simulink model "exercises_check"  (R2024a)
settings: Solver=FixedStepAuto  StartTime=0.0  StopTime=100  FixedStep=0.0001  MaxStep=1e-4  RelTol=1e-6
settings Model: Creator=kit  LastModifiedBy=kit

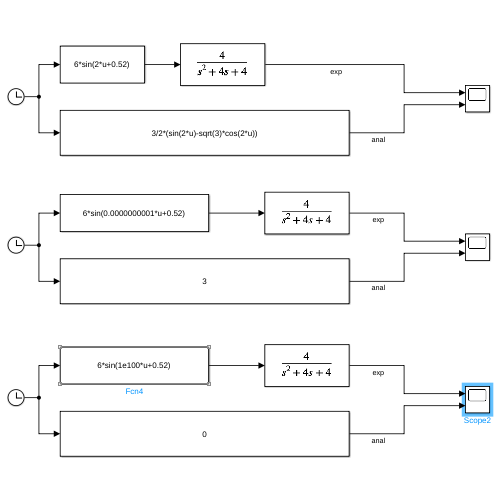
[thumbnail: Simulink's stored preview of the top-level diagram]
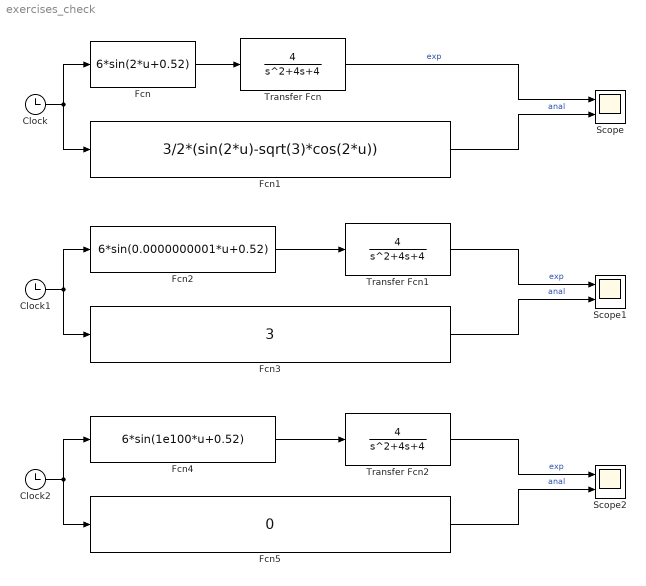
== system exercises_check ==
  Clock : Clock
  Clock1 : Clock
  Clock2 : Clock
  Fcn : Fcn  Expr=6*sin(2*u+0.52)
  Fcn1 : Fcn  Expr=3/2*(sin(2*u)-sqrt(3)*cos(2*u))
  Fcn2 : Fcn  Expr=6*sin(0.0000000001*u+0.52)
  Fcn3 : Fcn  Expr=3
  Fcn4 : Fcn  Expr=6*sin(1e100*u+0.52)
  Fcn5 : Fcn  Expr=0
  Scope : Scope  NumInputPorts=2
  Scope1 : Scope  NumInputPorts=2
  Scope2 : Scope  NumInputPorts=2
  Transfer Fcn : TransferFcn  Numerator=[4]  Denominator=[1 4 4]
  Transfer Fcn1 : TransferFcn  Numerator=[4]  Denominator=[1 4 4]
  Transfer Fcn2 : TransferFcn  Numerator=[4]  Denominator=[1 4 4]
  wires:
  Clock/1 -> Fcn/1, Fcn1/1
  Fcn/1 -> Transfer Fcn/1
  Transfer Fcn/1 -> Scope/1  "exp"
  Fcn1/1 -> Scope/2  "anal"
  Clock1/1 -> Fcn2/1, Fcn3/1
  Fcn2/1 -> Transfer Fcn1/1
  Transfer Fcn1/1 -> Scope1/1  "exp"
  Fcn3/1 -> Scope1/2  "anal"
  Clock2/1 -> Fcn4/1, Fcn5/1
  Fcn4/1 -> Transfer Fcn2/1
  Transfer Fcn2/1 -> Scope2/1  "exp"
  Fcn5/1 -> Scope2/2  "anal"
